simulink library "bayesianAscent2_cl"  (R2018b)
settings: Solver=VariableStepAuto  StartTime=0.0  StopTime=10.0  RelTol=1e-3
settings Model: Creator=Ayaz  LastModifiedBy=Ayaz

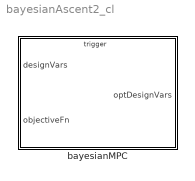
== system bayesianAscent2_cl ==
  bayesianMPC : Subsystem  TreatAsAtomicUnit=on  mask{gpModel=0, gpTrain=0, gpTrainFval=0, desLims=0, gamma=0.01, beta=1.1, iniTauPerc=0.1, maxIter=1, predHorz=1, ctrlHorz=1}
      mask prompts: gpModel "Gaussian process class"; gpTrain "Training desgin set"; gpTrainFval "Training objective function values"; desLims "Design limits"; iniTauPerc "Initial tau percentage"; maxIter "Max iterations"; predHorz "MPC prediction horizon"; ctrlHorz "MPC control horizon"

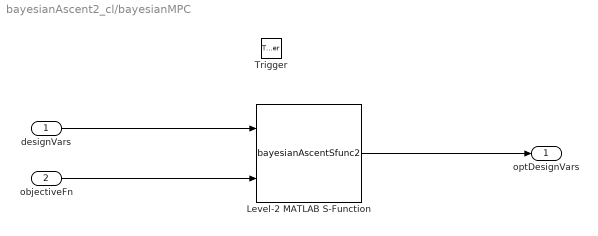
== system bayesianAscent2_cl/bayesianMPC ==
  designVars : Inport
  objectiveFn : Inport  Port=2
  Trigger : TriggerPort  VariantControl=Variant  InitialTriggerSignalState=zero
  Level-2 MATLAB S-Function : M-S-Function  FunctionName=bayesianAscentSfunc2  Parameters=gpTrain,gpTrainFval,desLims,gamma,beta,iniTauPerc,maxIter,gpModel,predHorz,ctrlHorz
  optDesignVars : Outport
  wires:
  designVars/1 -> Level-2 MATLAB S-Function/1
  objectiveFn/1 -> Level-2 MATLAB S-Function/2
  Level-2 MATLAB S-Function/1 -> optDesignVars/1
